simulink model "Main_model"  (R2018a)
settings: Solver=VariableStepAuto  StartTime=0.0  StopTime=0.04  MaxStep=1e-7  RelTol=1e-5
values from neighbouring files (symbols this model uses):
  M = 10^6*M    [design_code.m]
undefined symbols (not defined in the file or in its folder): fop, Ip_peak, R, Vin_peak
libraries: powerlib x69, powerlib_meascontrol x3, simulink x2
settings Model: Creator=user  LastModifiedBy=user

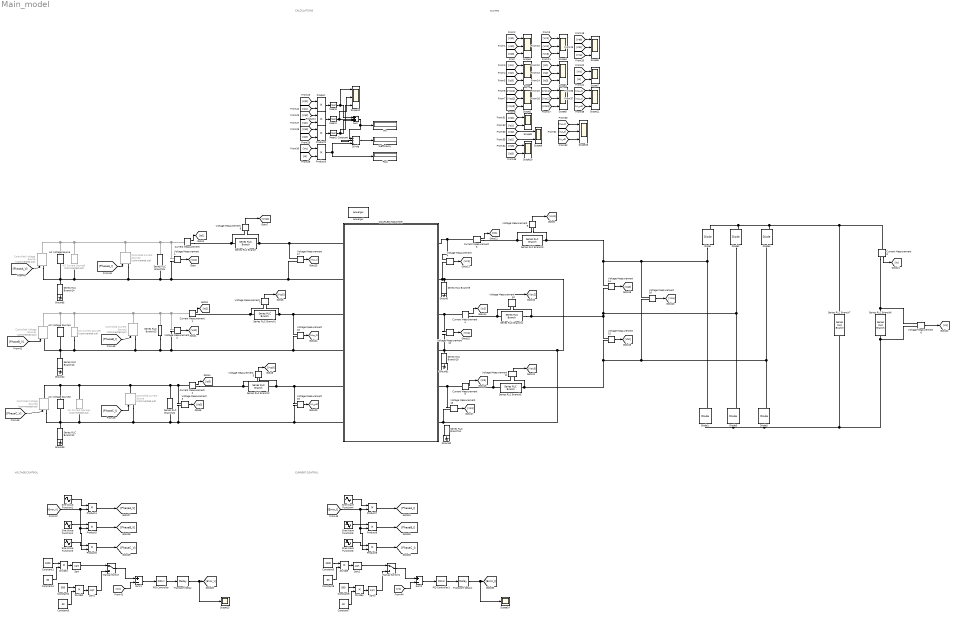
== system Main_model ==
  note: VOLTAGE CONTROL
  note: CALCULATIONS
  note: SCOPES
  note: CURRENT CONTROL
  %Efficiency : Display
  AC Current Source4 : powerlib/Electrical Sources/AC Current Source  Commented=on  Amplitude=Ip_peak  Phase=240  Frequency=fop*1e3  SampleTime=0  Measurements=None
      settings: SourceProductName=Simscape Power Systems  SourceProductBaseCode=PS
  AC Current Source5 : powerlib/Electrical Sources/AC Current Source  Commented=on  Amplitude=Ip_peak  Phase=0  Frequency=fop*1e3  SampleTime=0  Measurements=None
      settings: SourceProductName=Simscape Power Systems  SourceProductBaseCode=PS
  AC Current Source6 : powerlib/Electrical Sources/AC Current Source  Commented=on  Amplitude=Ip_peak  Phase=0  Frequency=fop*1e3  SampleTime=0  Measurements=None
      settings: SourceProductName=Simscape Power Systems  SourceProductBaseCode=PS
  AC Voltage Source : powerlib/Electrical Sources/AC Voltage Source  Amplitude=Vin_peak  Phase=0  Frequency=fop*1e3  SampleTime=0  Measurements=None  BusType=swing  Pref=10e3  Qref=0  Qmin=-inf  Qmax=+inf
  AC Voltage Source1 : powerlib/Electrical Sources/AC Voltage Source  Amplitude=Vin_peak  Phase=120  Frequency=fop*1e3  SampleTime=0  Measurements=None  BusType=swing  Pref=10e3  Qref=0  Qmin=-inf  Qmax=+inf
  AC Voltage Source2 : powerlib/Electrical Sources/AC Voltage Source  Amplitude=Vin_peak  Phase=240  Frequency=fop*1e3  SampleTime=0  Measurements=None  BusType=swing  Pref=10e3  Qref=0  Qmin=-inf  Qmax=+inf
  COUPLED INDUCTOR : Subsystem
  Constant : Constant  Value=100
  Constant1 : Constant  Value=1000
  Constant2 : Constant  Value=500
  Constant{3..4,7..8} (4 alike) : Constant  Value=30
  Constant5 : Constant  Value=1000
  Constant6 : Constant  Value=500
  Controlled Current Source : powerlib/Electrical Sources/Controlled Current Source  Commented=on  Initialize=on  Source_Type=AC  Amplitude=0  Phase=0  Frequency=0  Measurements=None
  Controlled Current Source1 : powerlib/Electrical Sources/Controlled Current Source  Commented=on  Initialize=on  Source_Type=AC  Amplitude=0  Phase=0  Frequency=0  Measurements=None
  Controlled Current Source2 : powerlib/Electrical Sources/Controlled Current Source  Commented=on  Initialize=on  Source_Type=AC  Amplitude=0  Phase=0  Frequency=0  Measurements=None
  Controlled Voltage Source : powerlib/Electrical Sources/Controlled Voltage Source  Commented=on  Initialize=on  Source_Type=AC  Amplitude=0  Phase=0  Frequency=0  Measurements=None
  Controlled Voltage Source1 : powerlib/Electrical Sources/Controlled Voltage Source  Commented=on  Initialize=on  Source_Type=AC  Amplitude=0  Phase=0  Frequency=0  Measurements=None
  Controlled Voltage Source2 : powerlib/Electrical Sources/Controlled Voltage Source  Commented=on  Initialize=on  Source_Type=AC  Amplitude=0  Phase=0  Frequency=0  Measurements=None
  Current Measurement{,1..6} (7 alike) : powerlib/Measurements/Current Measurement  PhasorSimulation=off  OutputType=Complex  PSBequivalent=0
  Diode{,1..5} (6 alike) : powerlib/Power Electronics/Diode  Ron=0.001  Lon=0  Vf=0.8  IC=0  UseSnubber=0  Rs=inf  Cs=250e-9  Measurements=on
  Divide : Product  Inputs=/**
  Divide{1..4} (4 alike) : Product  Inputs=**
  Ground{,1..5} (6 alike) : powerlib/Elements/Ground  LConnTagsString=a
  Manual Switch : ManualSwitch
  Manual Switch1 : ManualSwitch
  Mean1 : powerlib_meascontrol/Measurements/Mean  Freq=fop*2e3  Vinit=0  Ts=0
  Mean2 : powerlib_meascontrol/Measurements/Mean  Freq=fop*2e3  Vinit=0  Ts=0
  Mean3 : powerlib_meascontrol/Measurements/Mean  Freq=fop*2e3  Vinit=0  Ts=0
  PID Controller : simulink/Continuous/PID Controller  Controller=PID  TimeDomain=Continuous-time  SampleTime=-1  IntegratorMethod=Forward Euler  FilterMethod=Forward Euler  Form=Parallel  UseFilter=on  ControllerParametersSource=internal  P=0.1  I=10000  D=0  N=100  InitialConditionSource=internal  InitialConditionForIntegrator=0  InitialConditionForFilter=0  ExternalReset=none  LimitOutput=on  UpperSaturationLimit=inf  LowerSaturationLimit=-inf  LinearizeAsGain=on  AntiWindupMode=clamping  Kb=1  TrackingMode=off  Kt=1  PParamMin=[]  PParamMax=[]  IParamMin=[]  IParamMax=[]  DParamMin=[]  DParamMax=[]  NParamMin=[]  NParamMax=[]  KbParamMin=[]  KbParamMax=[]  KtParamMin=[]  KtParamMax=[]  POutMin=[]  POutMax=[]  IOutMin=[]  IOutMax=[]  DOutMin=[]  DOutMax=[]  NOutMin=[]  NOutMax=[]  KbOutMin=[]  KbOutMax=[]  KtOutMin=[]  KtOutMax=[]  IntegratorOutMin=[]  IntegratorOutMax=[]  FilterOutMin=[]  FilterOutMax=[]  SumOutMin=[]  SumOutMax=[]  SumI1OutMin=[]  SumI1OutMax=[]  SumI2OutMin=[]  SumI2OutMax=[]  SumI3OutMin=[]  SumI3OutMax=[]  SumDOutMin=[]  SumDOutMax=[]  SaturationOutMin=[]  SaturationOutMax=[]  IntegratorContinuousStateAttributes=''  IntegratorStateMustResolveToSignalObject=off  IntegratorRTWStateStorageClass=Auto  FilterContinuousStateAttributes=''  FilterStateMustResolveToSignalObject=off  FilterRTWStateStorageClass=Auto  DifferentiatorICPrevScaledInput=0  DifferentiatorOutMin=[]  DifferentiatorOutMax=[]  FilterDiffOutCoefMin=[]  FilterDiffOutCoefMax=[]  SumDenOutMin=[]  SumDenOutMax=[]  SumNumOutMin=[]  SumNumOutMax=[]  ReciprocalOutMin=[]  ReciprocalOutMax=[]  DivideOutMin=[]  DivideOutMax=[]  TunerSelectOption=Transfer Function Based (PID Tuner App)
  PID Controller1 : simulink/Continuous/PID Controller  Controller=PID  TimeDomain=Continuous-time  SampleTime=-1  IntegratorMethod=Forward Euler  FilterMethod=Forward Euler  Form=Parallel  UseFilter=on  ControllerParametersSource=internal  P=0.0038  I=800  D=0  N=100  InitialConditionSource=internal  InitialConditionForIntegrator=0  InitialConditionForFilter=0  ExternalReset=none  LimitOutput=on  UpperSaturationLimit=inf  LowerSaturationLimit=-inf  LinearizeAsGain=on  AntiWindupMode=clamping  Kb=1  TrackingMode=off  Kt=1  PParamMin=[]  PParamMax=[]  IParamMin=[]  IParamMax=[]  DParamMin=[]  DParamMax=[]  NParamMin=[]  NParamMax=[]  KbParamMin=[]  KbParamMax=[]  KtParamMin=[]  KtParamMax=[]  POutMin=[]  POutMax=[]  IOutMin=[]  IOutMax=[]  DOutMin=[]  DOutMax=[]  NOutMin=[]  NOutMax=[]  KbOutMin=[]  KbOutMax=[]  KtOutMin=[]  KtOutMax=[]  IntegratorOutMin=[]  IntegratorOutMax=[]  FilterOutMin=[]  FilterOutMax=[]  SumOutMin=[]  SumOutMax=[]  SumI1OutMin=[]  SumI1OutMax=[]  SumI2OutMin=[]  SumI2OutMax=[]  SumI3OutMin=[]  SumI3OutMax=[]  SumDOutMin=[]  SumDOutMax=[]  SaturationOutMin=[]  SaturationOutMax=[]  IntegratorContinuousStateAttributes=''  IntegratorStateMustResolveToSignalObject=off  IntegratorRTWStateStorageClass=Auto  FilterContinuousStateAttributes=''  FilterStateMustResolveToSignalObject=off  FilterRTWStateStorageClass=Auto  DifferentiatorICPrevScaledInput=0  DifferentiatorOutMin=[]  DifferentiatorOutMax=[]  FilterDiffOutCoefMin=[]  FilterDiffOutCoefMax=[]  SumDenOutMin=[]  SumDenOutMax=[]  SumNumOutMin=[]  SumNumOutMax=[]  ReciprocalOutMin=[]  ReciprocalOutMax=[]  DivideOutMin=[]  DivideOutMax=[]  TunerSelectOption=Transfer Function Based (PID Tuner App)
  Pin : Display
  Pout : Display
  Product{,1..9} (10 alike) : Product
  Scope{,1..6,11..12,15} (10 alike) : Scope  NumInputPorts=3
  Scope{7..10} (4 alike) : Scope  NumInputPorts=2
  Scope13 : Scope
  Scope14 : Scope
  Series RLC Branch : powerlib/Elements/Series RLC Branch  LConnTagsString=__new0  RConnTagsString=__new0  BranchType=C  Resistance=1  Inductance=1e-3  SetiL0=off  InitialCurrent=0  Capacitance=7.7e-9  Setx0=off  InitialVoltage=0  Measurements=None
  Series RLC Branch1 : powerlib/Elements/Series RLC Branch  LConnTagsString=__new0  RConnTagsString=__new0  BranchType=C  Resistance=1  Inductance=1e-3  SetiL0=off  InitialCurrent=0  Capacitance=7.7e-9  Setx0=off  InitialVoltage=0  Measurements=None
  Series RLC Branch{9..14,22..24} (9 alike) : powerlib/Elements/Series RLC Branch  LConnTagsString=__new0  RConnTagsString=__new0  BranchType=R  Resistance=10000  Inductance=1e-3  SetiL0=off  InitialCurrent=0  Capacitance=9.95e-9  Setx0=off  InitialVoltage=0  Measurements=None
  Series RLC Branch2 : powerlib/Elements/Series RLC Branch  LConnTagsString=__new0  RConnTagsString=__new0  BranchType=C  Resistance=1  Inductance=1e-3  SetiL0=off  InitialCurrent=0  Capacitance=7.7e-9  Setx0=off  InitialVoltage=0  Measurements=None
  Series RLC Branch3 : powerlib/Elements/Series RLC Branch  LConnTagsString=__new0  RConnTagsString=__new0  BranchType=C  Resistance=1  Inductance=1e-3  SetiL0=off  InitialCurrent=0  Capacitance=9.95e-9  Setx0=off  InitialVoltage=0  Measurements=None
  Series RLC Branch4 : powerlib/Elements/Series RLC Branch  LConnTagsString=__new0  RConnTagsString=__new0  BranchType=C  Resistance=1  Inductance=1e-3  SetiL0=off  InitialCurrent=0  Capacitance=9.95e-9  Setx0=off  InitialVoltage=0  Measurements=None
  Series RLC Branch5 : powerlib/Elements/Series RLC Branch  LConnTagsString=__new0  RConnTagsString=__new0  BranchType=C  Resistance=1  Inductance=1e-3  SetiL0=off  InitialCurrent=0  Capacitance=9.95e-9  Setx0=off  InitialVoltage=0  Measurements=None
  Series RLC Branch6 : powerlib/Elements/Series RLC Branch  LConnTagsString=__new0  RConnTagsString=__new0  BranchType=R  Resistance=35  Inductance=1e-3  SetiL0=off  InitialCurrent=0  Capacitance=9.95e-9  Setx0=off  InitialVoltage=0  Measurements=None
  Series RLC Branch7 : powerlib/Elements/Series RLC Branch  LConnTagsString=__new0  RConnTagsString=__new0  BranchType=C  Resistance=30  Inductance=1e-3  SetiL0=off  InitialCurrent=0  Capacitance=1e-6  Setx0=off  InitialVoltage=0  Measurements=None
  Sine Wave Function1 : Sin  Frequency=fop*2*pi*1e3  SampleTime=0
  Sine Wave Function2 : Sin  Frequency=fop*2*pi*1e3  Phase=2*pi/3  SampleTime=0
  Sine Wave Function3 : Sin  Frequency=fop*2*pi*1e3  Phase=4*pi/3  SampleTime=0
  Sine Wave Function4 : Sin  Frequency=fop*2*pi*1e3  SampleTime=0
  Sine Wave Function5 : Sin  Frequency=fop*2*pi*1e3  Phase=2*pi/3  SampleTime=0
  Sine Wave Function6 : Sin  Frequency=fop*2*pi*1e3  Phase=4*pi/3  SampleTime=0
  Sqrt{,1..3} (4 alike) : Sqrt  SaturateOnIntegerOverflow=on
  Sum : Sum  Inputs=+++
  Sum1 : Sum  Inputs=+-
  Sum2 : Sum  Inputs=+-
  Transport Delay : TransportDelay  DelayTime=1e-6
  Transport Delay1 : TransportDelay  DelayTime=1e-6
  Voltage Measurement{1..19} (19 alike) : powerlib/Measurements/Voltage Measurement  PhasorSimulation=off  OutputType=Complex  PSBequivalent=0
  powergui : powerlib/powergui  Priority=1  SimulationMode=Continuous  SampleTime=50e-6  frequency=60  Iterations=50  frequencyindice=0  Pbase=100e6  ErrMax=1e-4  UnitsV=kV  UnitsW=MW  buscounter=0  FunctionMessages=off  echomessages=off  EnableUseOfTLC=off  CurrentSourceSwitches=off  DisableSnubberDevices=off  DisableRonSwitches=off  DisableVfSwitches=off  DisplayEquations=off  SolverType=Tustin/Backward Euler (TBE)  Interpol=off  ExternalGateDelay=off  methode=off  Ts=100  x0status=blocks  SPID=on  SwTol=0  HookPort=off  RestoreLinks=warning  ResistiveCurrentMeasurement=off  Frange=[0:2:500]  Ylog=off  Xlog=on  ShowGrid=off  save=off  variable=ZData  structure=0  ZoomFFT=off  StartTime=0.0  cycles=1  DisplayStyle=1  fundamental=60  FreqAxis=off  MaxFrequency=1000  frequencyindicesteady=1  RmsSteady=1  display=off
  wires:
  Voltage Measurement6/1 -> [Vo]
  Voltage Measurement1/1 -> [Vp1]
  Voltage Measurement2/1 -> [Vp2]
  Current Measurement/1 -> [Ip1]
  Current Measurement1/1 -> [Ip2]
  Current Measurement2/1 -> [Ip3]
  Voltage Measurement3/1 -> [Vp3]
  Voltage Measurement7/1 -> [Vcp2]
  Voltage Measurement8/1 -> [Vcp1]
  Voltage Measurement5/1 -> [Vcp3]
  Voltage Measurement9/1 -> [Vsc1]
  Voltage Measurement10/1 -> [Vsc2]
  Voltage Measurement11/1 -> [Vsc3]
  Current Measurement5/1 -> [Is1]
  Voltage Measurement4/1 -> [Vs1]
  Current Measurement4/1 -> [Is2]
  Voltage Measurement12/1 -> [Vs2]
  Current Measurement3/1 -> [Is3]
  Voltage Measurement13/1 -> [Vs3]
  Voltage Measurement14/1 -> [Vab]
  Voltage Measurement15/1 -> [Vbc]
  Voltage Measurement16/1 -> [Vca]
  Current Measurement6/1 -> [Io]
  [Ip1] -> Scope/1
  [Ip2] -> Scope/2
  [Ip3] -> Scope/3
  [Vp1] -> Scope1/1
  [Vp2] -> Scope1/2
  [Vp3] -> Scope1/3
  [Vcp1] -> Scope2/1
  [Vcp2] -> Scope2/2
  [Vcp3] -> Scope2/3
  [Vs1] -> Scope3/1
  [Vs2] -> Scope3/2
  [Vs3] -> Scope3/3
  [Is1] -> Scope4/1
  [Is2] -> Scope4/2
  [Is3] -> Scope4/3
  [Vsc1] -> Scope5/1
  [Vsc2] -> Scope5/2
  [Vsc3] -> Scope5/3
  [Vab] -> Scope6/1
  [Vbc] -> Scope6/2
  [Vca] -> Scope6/3
  [Vo] -> Scope7/1
  [Io] -> Scope7/2
  [Vp1] -> Product/1
  [Ip1] -> Product/2
  [Ip2] -> Product1/2
  [Vp2] -> Product1/1
  [Vp3] -> Product2/1
  [Ip3] -> Product2/2
  Product/1 -> Mean3/1
  Product1/1 -> Mean1/1
  Product2/1 -> Mean2/1
  Mean3/1 -> Scope12/1, Sum/1
  Mean1/1 -> Scope12/2, Sum/2
  Mean2/1 -> Scope12/3, Sum/3
  Sum/1 -> Divide/1, Pin/1
  [Io] -> Product3/2
  [Vo] -> Product3/1
  Product3/1 -> Pout/1, Divide/3
  Constant/1 -> Divide/2
  Divide/1 -> %Efficiency/1
  [Vp1] -> Scope8/1
  [Ip1] -> Scope8/2
  [Ip2] -> Scope9/2
  [Vp2] -> Scope9/1
  [Vp3] -> Scope10/1
  [Ip3] -> Scope10/2
  Voltage Measurement19/1 -> [VL_p3]
  Voltage Measurement18/1 -> [VLp_2]
  Voltage Measurement17/1 -> [VLp_1]
  [VLp_2] -> Scope11/1
  [VLp_1] -> Scope11/2
  [VL_p3] -> Scope11/3
  Transport Delay/1 -> Scope13/1, [Error_V]
  [PhaseA_V] -> Controlled Voltage Source/1
  [PhaseB_V] -> Controlled Voltage Source1/1
  [PhaseC_V] -> Controlled Voltage Source2/1
  Sine Wave Function1/1 -> Product4/1
  Sine Wave Function2/1 -> Product5/1
  Sine Wave Function3/1 -> Product6/1
  [Error_V] -> Product4/2, Product6/2, Product5/2
  Product4/1 -> [PhaseA_V]
  Product5/1 -> [PhaseB_V]
  Product6/1 -> [PhaseC_V]
  Manual Switch/1 -> Sum1/1
  [Vo] -> Sum1/2
  Sqrt/1 -> Manual Switch/1
  PID Controller/1 -> Transport Delay/1
  Sum1/1 -> PID Controller/1
  Constant1/1 -> Divide1/1
  Constant4/1 -> Divide1/2
  Divide1/1 -> Sqrt/1
  Divide2/1 -> Sqrt1/1
  Constant3/1 -> Divide2/2
  Constant2/1 -> Divide2/1
  Sqrt1/1 -> Manual Switch/2
  Sqrt3/1 -> Manual Switch1/2
  Constant6/1 -> Divide4/1
  Constant7/1 -> Divide4/2
  Divide4/1 -> Sqrt3/1
  Divide3/1 -> Sqrt2/1
  Constant8/1 -> Divide3/2
  Constant5/1 -> Divide3/1
  Sum2/1 -> PID Controller1/1
  PID Controller1/1 -> Transport Delay1/1
  Sqrt2/1 -> Manual Switch1/1
  [Vo] -> Sum2/2
  Manual Switch1/1 -> Sum2/1
  Product9/1 -> [PhaseC_I]
  Product8/1 -> [PhaseB_I]
  Product7/1 -> [PhaseA_I]
  [Error_I] -> Product8/2, Product9/2, Product7/2
  Sine Wave Function6/1 -> Product9/1
  Sine Wave Function5/1 -> Product8/1
  Sine Wave Function4/1 -> Product7/1
  Transport Delay1/1 -> [Error_I], Scope14/1
  [PhaseA_I] -> Controlled Current Source2/1
  [PhaseB_I] -> Controlled Current Source1/1
  [PhaseC_I] -> Controlled Current Source/1
  [VLp_2] -> Scope15/2
  [VLp_1] -> Scope15/1
  [VL_p3] -> Scope15/3
  connections:
  Diode2/LConn1 -- Diode3/RConn1 -- Voltage Measurement10/LConn2 -- Series RLC Branch4/RConn1 -- Voltage Measurement15/LConn1 -- Voltage Measurement14/LConn2
  Diode5/RConn1 -- Voltage Measurement16/LConn2 -- Voltage Measurement15/LConn2 -- Voltage Measurement11/LConn2 -- Series RLC Branch5/RConn1 -- Diode4/LConn1
  COUPLED INDUCTOR/LConn6 -- Voltage Measurement12/LConn2 -- Series RLC Branch10/LConn1 -- COUPLED INDUCTOR/LConn4 -- COUPLED INDUCTOR/LConn2 -- Voltage Measurement4/LConn2 -- Series RLC Branch9/LConn1 -- Voltage Measurement13/LConn2
  Diode4/RConn1 -- Current Measurement6/LConn1 -- Series RLC Branch7/LConn1 -- Diode/RConn1 -- Diode2/RConn1
  Diode/LConn1 -- Voltage Measurement16/LConn1 -- Voltage Measurement14/LConn1 -- Voltage Measurement9/LConn2 -- Series RLC Branch3/RConn1 -- Diode1/RConn1
  Diode3/LConn1 -- Diode1/LConn1 -- Series RLC Branch7/RConn1 -- Voltage Measurement6/LConn2 -- Series RLC Branch6/RConn1 -- Diode5/LConn1
  AC Voltage Source1/LConn1 -- Controlled Voltage Source1/LConn1 -- Controlled Current Source1/LConn1 -- Voltage Measurement18/LConn2 -- COUPLED INDUCTOR/RConn4 -- Voltage Measurement2/LConn2 -- Series RLC Branch23/RConn1 -- AC Current Source5/LConn1 -- Series RLC Branch13/LConn1
  Current Measurement5/RConn1 -- Voltage Measurement9/LConn1 -- Series RLC Branch3/LConn1
  Current Measurement2/LConn1 -- Voltage Measurement3/LConn1 -- AC Current Source4/RConn1 -- Controlled Voltage Source2/RConn1 -- AC Voltage Source2/RConn1 -- Controlled Current Source/RConn1 -- Series RLC Branch22/LConn1
  AC Current Source5/RConn1 -- Controlled Current Source1/RConn1 -- Series RLC Branch23/LConn1 -- Voltage Measurement2/LConn1 -- Current Measurement1/LConn1 -- Controlled Voltage Source1/RConn1 -- AC Voltage Source1/RConn1
  AC Current Source6/RConn1 -- Controlled Current Source2/RConn1 -- Series RLC Branch24/LConn1 -- Voltage Measurement1/LConn1 -- Current Measurement/LConn1 -- Controlled Voltage Source/RConn1 -- AC Voltage Source/RConn1
  Current Measurement4/LConn1 -- Voltage Measurement12/LConn1 -- COUPLED INDUCTOR/LConn3
  Current Measurement2/RConn1 -- Voltage Measurement5/LConn1 -- Series RLC Branch2/LConn1
  Current Measurement5/LConn1 -- Voltage Measurement4/LConn1 -- COUPLED INDUCTOR/LConn1
  Current Measurement4/RConn1 -- Voltage Measurement10/LConn1 -- Series RLC Branch4/LConn1
  Current Measurement3/LConn1 -- Voltage Measurement13/LConn1 -- COUPLED INDUCTOR/LConn5
  Current Measurement/RConn1 -- Voltage Measurement8/LConn1 -- Series RLC Branch/LConn1
  COUPLED INDUCTOR/RConn3 -- Voltage Measurement18/LConn1 -- Voltage Measurement7/LConn2 -- Series RLC Branch1/RConn1
  COUPLED INDUCTOR/RConn1 -- Voltage Measurement17/LConn1 -- Voltage Measurement8/LConn2 -- Series RLC Branch/RConn1
  COUPLED INDUCTOR/RConn5 -- Voltage Measurement19/LConn1 -- Voltage Measurement5/LConn2 -- Series RLC Branch2/RConn1
  Current Measurement1/RConn1 -- Voltage Measurement7/LConn1 -- Series RLC Branch1/LConn1
  Series RLC Branch5/LConn1 -- Voltage Measurement11/LConn1 -- Current Measurement3/RConn1
  Series RLC Branch14/LConn1 -- Controlled Voltage Source/LConn1 -- Controlled Current Source2/LConn1 -- Voltage Measurement17/LConn2 -- COUPLED INDUCTOR/RConn2 -- Voltage Measurement1/LConn2 -- Series RLC Branch24/RConn1 -- AC Current Source6/LConn1 -- AC Voltage Source/LConn1
  Series RLC Branch12/LConn1 -- Controlled Voltage Source2/LConn1 -- AC Current Source4/LConn1 -- Voltage Measurement19/LConn2 -- COUPLED INDUCTOR/RConn6 -- Voltage Measurement3/LConn2 -- Series RLC Branch22/RConn1 -- Controlled Current Source/LConn1 -- AC Voltage Source2/LConn1
  Series RLC Branch6/LConn1 -- Current Measurement6/RConn1 -- Voltage Measurement6/LConn1

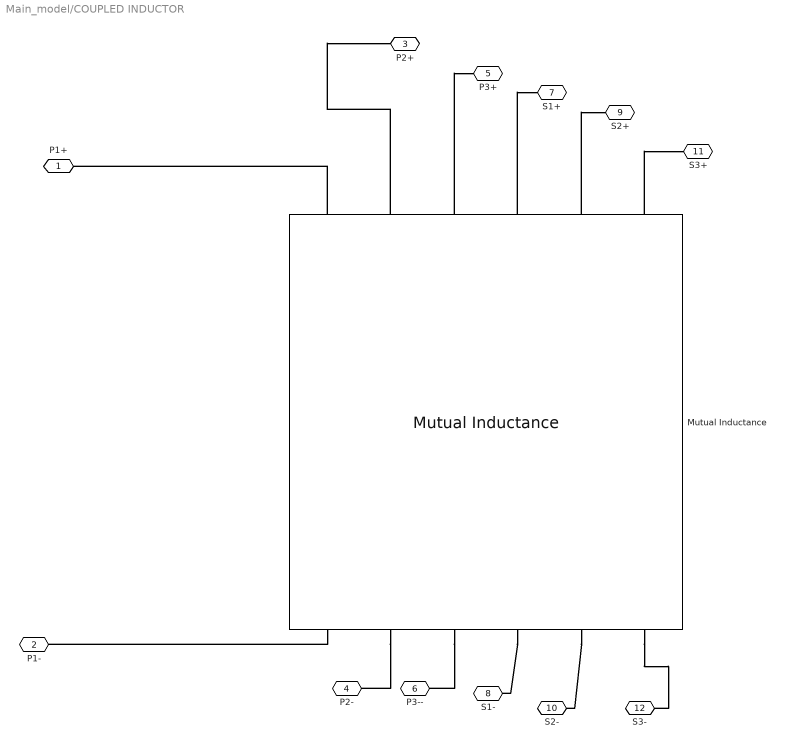
== system Main_model/COUPLED INDUCTOR ==
  Mutual Inductance : powerlib/Elements/Mutual Inductance  LConnTagsString=a|b|c|L4|L5|L6  RConnTagsString=A|B|C|R4|R5|R6  TypeOfMutual=Generalized mutual inductance  NumberOfWindings=6  SelfImpedance1=[1.1 1.1e-03]  SelfImpedance2=[ 1.1 1.1e-03]  ThreeWindings=on  SelfImpedance3=[ 1.1 1.1e-03]  MutualImpedance=[1.0 1.0e-03]  InductanceMatrix=M * 1e-6  ResistanceMatrix=R*0.001  Measurements=None
      settings: AttributesFormatString=\n  SourceProductName=Simscape Power Systems  SourceProductBaseCode=PS
  P1+ : PMIOPort  Side=Right
  P1- : PMIOPort  Port=2  Side=Right
  P2+ : PMIOPort  Port=3  Side=Right
  P2- : PMIOPort  Port=4  Side=Right
  P3+ : PMIOPort  Port=5  Side=Right
  P3-- : PMIOPort  Port=6  Side=Right
  S1+ : PMIOPort  Port=7  Side=Left
  S1- : PMIOPort  Port=8  Side=Left
  S2+ : PMIOPort  Port=9  Side=Left
  S2- : PMIOPort  Port=10  Side=Left
  "S3+ " : PMIOPort  Port=11  Side=Left
  "S3- " : PMIOPort  Port=12  Side=Left
  connections:
  Mutual Inductance/LConn2 -- P2-/RConn1
  Mutual Inductance/LConn5 -- S2-/RConn1
  Mutual Inductance/RConn5 -- S2+/RConn1
  Mutual Inductance/RConn4 -- S1+/RConn1
  Mutual Inductance/LConn6 -- "S3- "/RConn1
  Mutual Inductance/RConn1 -- P1+/RConn1
  Mutual Inductance/LConn1 -- P1-/RConn1
  Mutual Inductance/RConn2 -- P2+/RConn1
  Mutual Inductance/LConn4 -- S1-/RConn1
  Mutual Inductance/LConn3 -- P3--/RConn1
  Mutual Inductance/RConn3 -- P3+/RConn1
  Mutual Inductance/RConn6 -- "S3+ "/RConn1
